simulink model "gm_flyback_dt"  (R2021b)
settings: Solver=FixedStepDiscrete  StartTime=0.0  StopTime=100e-3  RelTol=1e-3
undefined symbols (not defined in the file or in its folder): DiscIntNeverNeededParam
Description:
  | Symmetric FIR Filter
  | This example shows how to use HDL Coder(TM) to check, generate,
  | and verify HDL for a fixed-point symmetric FIR filter.
settings Model: Creator=The MathWorks, Inc.  LastModifiedBy=Marco Milanesi
settings SolverCC: AlgebraicLoopSolver=TrustRegion  AutoInsertRateTranBlk=on
settings DataIOCC: LimitDataPoints=on  SaveFormat=Array  SaveOutput=off  SignalLogging=off  SaveTime=off  ReturnWorkspaceOutputs=off  SignalLoggingName=logsOut
settings OptimizationCC: BlockReduction=off  BooleanDataType=off  ConditionallyExecuteInputs=off  DefaultParameterBehavior=Inlined  InheritOutputTypeSmallerThanSingle=on  InlineInvariantSignals=on  ExpressionDepthLimit=2147483647  InitFltsAndDblsToZero=on  LifeSpan=inf  BufferReusableBoundary=off
settings DebuggingCC: AlgebraicLoopMsg=error  SaveWithParameterizedLinksMsg=none  UnderspecifiedInitializationDetection=Classic  MergeDetectMultiDrivingBlocksExec=none  CheckExecutionContextPreStartOutputMsg=on  SignalResolutionControl=TryResolveAllWithWarning  InheritedTsInSrcMsg=none  MultiTaskDSMMsg=warning  MultiTaskCondExecSysMsg=none  SingleTaskRateTransMsg=error  IntegerOverflowMsg=none  ParameterPrecisionLossMsg=none  FcnCallInpInsideContextMsg=warning  BusObjectLabelMismatch=none  StateNameClashWarn=warning  SFUnexpectedBacktrackingDiag=warning  SFNoUnconditionalDefaultTransitionDiag=warning  SFExecutionAtInitializationDiag=none  SFMachineParentedDataDiag=warning  IntegerSaturationMsg=none  ArithmeticOperatorsInVariantConditions=warning
settings HardwareCC: ProdBitPerPointer=32  ProdBitPerSizeT=32  ProdBitPerPtrDiffT=32  ProdLargestAtomicFloat=None  ProdIntDivRoundTo=Undefined  ProdEndianess=Unspecified  ProdWordSize=32  ProdHWDeviceType=ASIC/FPGA  TargetUnknown=on  ProdEqTarget=off
settings ModelReferenceCC: PropagateSignalLabelsOutOfModel=off
settings SFSimCC: SimUseLocalCustomCode=off  CustomCodeUndefinedFunction=UseInterfaceOnly
settings RTWCC: RTWUseLocalCustomCode=off
settings CodeAppCC: StateflowObjectComments=on
settings GRTTargetCC: TargetFcnLib=ansi_tfl_tmw.mat  TargetLangStandard=C89/C90 (ANSI)  CombineOutputUpdateFcns=off  GRTInterface=on
settings ConfigComp: CovMetricSettings=dw  CovSaveCumulativeToWorkspaceVar=on  CovSaveSingleToWorkspaceVar=on  CovExternalEMLEnable=off

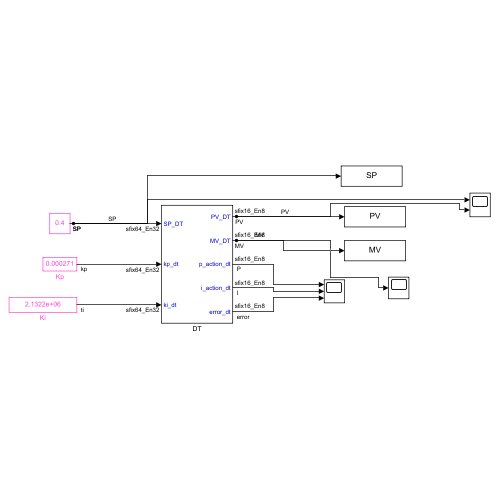
[thumbnail: Simulink's stored preview of the top-level diagram]
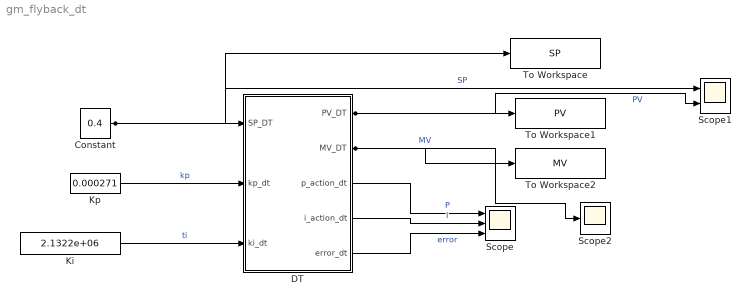
== system gm_flyback_dt ==
  Constant : Constant  Value=0.4  OutDataTypeStr=fixdt(1,64,32)
  DT : Subsystem
  Ki : Constant  Value=2.1322e+06  OutDataTypeStr=fixdt(1,64,32)
  Kp : Constant  Value=0.000271  OutDataTypeStr=fixdt(1,64,32)
  Scope : Scope  NumInputPorts=3
  Scope1 : Scope  NumInputPorts=2
  Scope2 : Scope
  To Workspace : ToWorkspace  VariableName=SP  SaveFormat=Structure With Time  SampleTime=-1
  To Workspace1 : ToWorkspace  VariableName=PV  SaveFormat=Structure With Time  SampleTime=-1
  To Workspace2 : ToWorkspace  VariableName=MV  SaveFormat=Structure With Time  SampleTime=-1
  wires:
  DT/4(i_action_dt) -> Scope/2  "I"
  DT/2(MV_DT) -> To Workspace2/1, Scope2/1  "MV"
  DT/1(PV_DT) -> To Workspace1/1, Scope1/2  "PV"
  DT/5(error_dt) -> Scope/3  "error"
  DT/3(p_action_dt) -> Scope/1  "P"
  Constant/1 -> DT/1(SP_DT), To Workspace/1, Scope1/1  "SP"
  Ki/1 -> DT/3(ki_dt)  "ti"
  Kp/1 -> DT/2(kp_dt)  "kp"

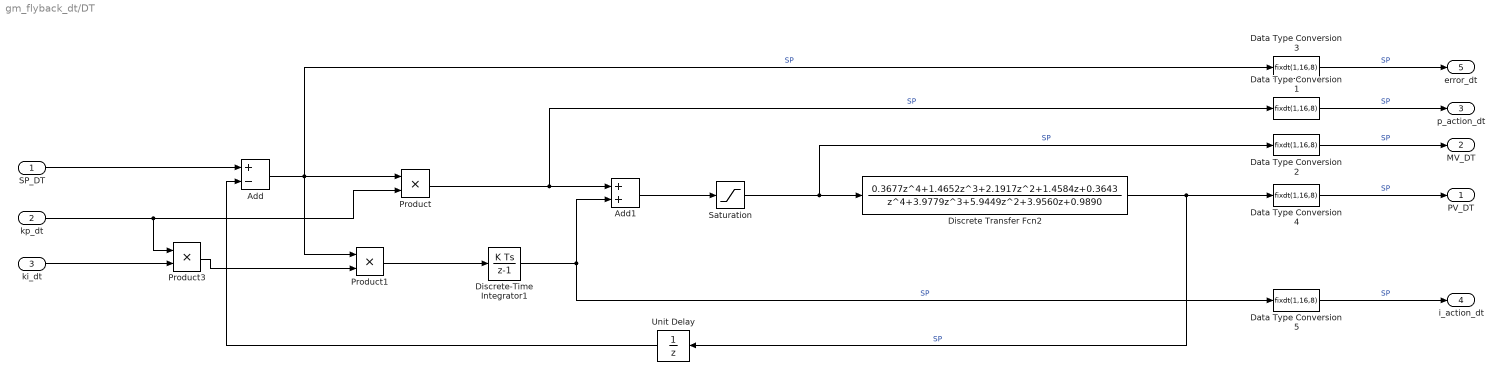
== system gm_flyback_dt/DT ==
  SP_DT : Inport  OutDataTypeStr=fixdt(1,64,32)  SampleTime=0.00001
  kp_dt : Inport  Port=2  OutDataTypeStr=fixdt(1,64,32)  SampleTime=0.00001
  ki_dt : Inport  Port=3  OutDataTypeStr=fixdt(1,64,32)  SampleTime=0.00001
  Add : Sum  Inputs=+-  AccumDataTypeStr=fixdt(1,64,32)  OutDataTypeStr=fixdt(1,64,32)
  Add1 : Sum  AccumDataTypeStr=fixdt(1,64,32)  OutDataTypeStr=fixdt(1,64,32)
  Data Type Conversion{1..5} (5 alike) : DataTypeConversion  OutDataTypeStr=fixdt(1,16,8)
  Discrete Transfer Fcn2 : DiscreteTransferFcn  Numerator=[0.3677 1.4652 2.1917 1.4584 0.3643]  Denominator=[1 3.9779 5.9449 3.9560 0.9890]  SampleTime=0.00001  NumCoefDataTypeStr=fixdt(1,64,32)  DenCoefDataTypeStr=fixdt(1,64,32)  NumProductDataTypeStr=fixdt(1,64,32)  DenProductDataTypeStr=fixdt(1,64,32)  NumAccumDataTypeStr=fixdt(1,64,32)  DenAccumDataTypeStr=fixdt(1,64,32)  OutDataTypeStr=fixdt(1,64,32)
  Discrete-Time Integrator1 : DiscreteIntegrator  SampleTime=0.00001  OutDataTypeStr=fixdt(1,64,32)  ICPrevOutput=DiscIntNeverNeededParam  ICPrevScaledInput=DiscIntNeverNeededParam
  Product : Product  OutDataTypeStr=fixdt(1,64,32)
  Product1 : Product  OutDataTypeStr=fixdt(1,64,32)
  Product3 : Product  OutDataTypeStr=fixdt(1,64,32)
  Saturation : Saturate  UpperLimit=10  LowerLimit=-10  OutDataTypeStr=fixdt(1,64,32)
  Unit Delay : UnitDelay  SampleTime=0.00001  HasFrameUpgradeWarning=on
  PV_DT : Outport  OutDataTypeStr=fixdt(1,16,8)  SampleTime=0.00001  VectorParamsAs1DForOutWhenUnconnected=off
  MV_DT : Outport  Port=2  OutDataTypeStr=fixdt(1,16,8)  SampleTime=0.00001  VectorParamsAs1DForOutWhenUnconnected=off
  p_action_dt : Outport  Port=3  OutDataTypeStr=fixdt(1,16,8)  SampleTime=0.00001  VectorParamsAs1DForOutWhenUnconnected=off
  i_action_dt : Outport  Port=4  OutDataTypeStr=fixdt(1,16,8)  SampleTime=0.00001  VectorParamsAs1DForOutWhenUnconnected=off
  error_dt : Outport  Port=5  OutDataTypeStr=fixdt(1,16,8)  SampleTime=0.00001  VectorParamsAs1DForOutWhenUnconnected=off
  wires:
  Data Type Conversion5/1 -> i_action_dt/1  "SP"
  Data Type Conversion4/1 -> PV_DT/1  "SP"
  Data Type Conversion2/1 -> MV_DT/1  "SP"
  Data Type Conversion3/1 -> error_dt/1  "SP"
  Data Type Conversion1/1 -> p_action_dt/1  "SP"
  Discrete-Time Integrator1/1 -> Add1/2, Data Type Conversion5/1  "SP"
  Saturation/1 -> Data Type Conversion2/1, Discrete Transfer Fcn2/1  "SP"
  Discrete Transfer Fcn2/1 -> Unit Delay/1, Data Type Conversion4/1  "SP"
  Product/1 -> Add1/1, Data Type Conversion1/1  "SP"
  Add/1 -> Product1/1, Product/1, Data Type Conversion3/1  "SP"
  Product3/1 -> Product1/2
  ki_dt/1 -> Product3/2
  Product1/1 -> Discrete-Time Integrator1/1
  Add1/1 -> Saturation/1
  Unit Delay/1 -> Add/2
  kp_dt/1 -> Product3/1, Product/2
  SP_DT/1 -> Add/1
